simulink model "Crazyflie_NoLinealModel"  (R2020b)
settings: Solver=VariableStepAuto  StartTime=0.0  StopTime=10.0  RelTol=1e-3
undefined symbols (not defined in the file): fm, g, Ixx, Iyy, Izz, m, MNL1
settings Model: Creator=FranciscoJose  LastModifiedBy=FranciscoJose

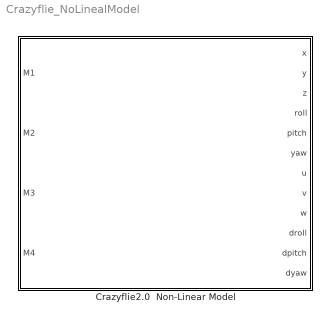
== system Crazyflie_NoLinealModel ==
  Crazyflie2.0  Non-Linear Model : Subsystem
      mask Display: image('crazyflie_icon.png')

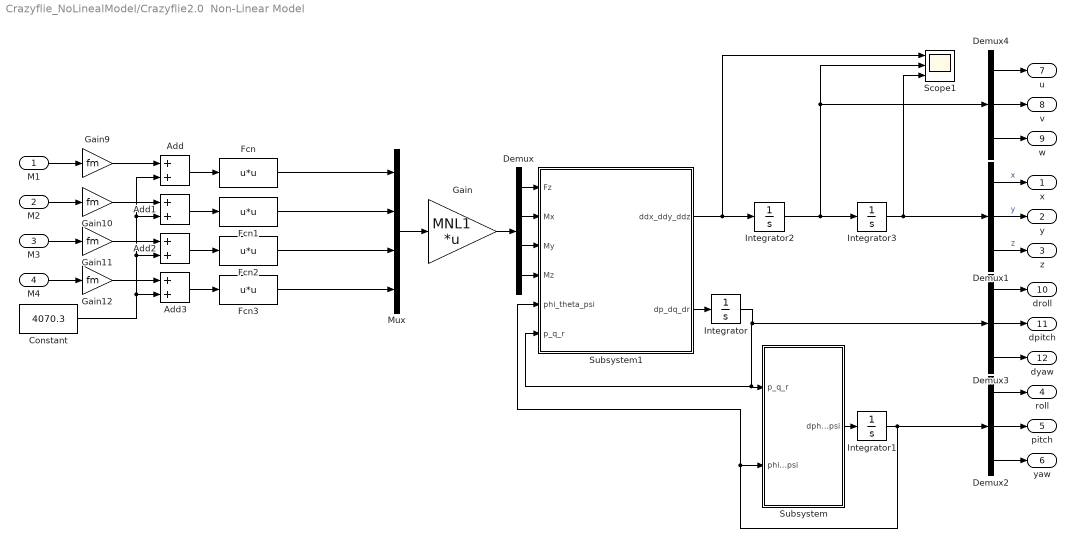
== system Crazyflie_NoLinealModel/Crazyflie2.0  Non-Linear Model ==
  M1 : Inport
  M2 : Inport  Port=2
  M3 : Inport  Port=3
  M4 : Inport  Port=4
  Add{,1..3} (4 alike) : Sum
  Constant : Constant  Value=4070.3
  Demux : Demux
  Demux{1..4} (4 alike) : Demux  Outputs=3
  Fcn{,1..3} (4 alike) : Fcn  Expr=u*u
  Gain : Gain  Gain=MNL1  Multiplication=Matrix(K*u) (u vector)
  Gain{9..12} (4 alike) : Gain  Gain=fm
  Integrator{,1..3} (4 alike) : Integrator
  Mux : Mux
  Scope1 : Scope  NumInputPorts=3
  Subsystem : Subsystem
  Subsystem1 : Subsystem
  x : Outport
  y : Outport  Port=2
  z : Outport  Port=3
  roll : Outport  Port=4
  pitch : Outport  Port=5
  yaw : Outport  Port=6
  u : Outport  Port=7
  v : Outport  Port=8
  w : Outport  Port=9
  droll : Outport  Port=10
  dpitch : Outport  Port=11
  dyaw : Outport  Port=12
  wires:
  Mux/1 -> Gain/1
  Gain/1 -> Demux/1
  Demux/1 -> Subsystem1/1(Fz)
  Demux/2 -> Subsystem1/2(Mx)
  Demux/3 -> Subsystem1/3(My)
  Demux/4 -> Subsystem1/4(Mz)
  Demux1/1 -> x/1  "x"
  Demux1/2 -> y/1  "y"
  Demux1/3 -> z/1  "z"
  Demux2/1 -> roll/1
  Demux2/2 -> pitch/1
  Demux2/3 -> yaw/1
  Demux4/1 -> u/1
  Demux4/2 -> v/1
  Demux4/3 -> w/1
  Demux3/1 -> droll/1
  Demux3/2 -> dpitch/1
  Demux3/3 -> dyaw/1
  M1/1 -> Gain9/1
  M2/1 -> Gain10/1
  M3/1 -> Gain11/1
  M4/1 -> Gain12/1
  Subsystem1/2(dp_dq_dr) -> Integrator/1
  Integrator/1 -> Demux3/1, Subsystem1/6(p_q_r), Subsystem/1(p_q_r)
  Subsystem/1(dphi_dtheta_dpsi) -> Integrator1/1
  Integrator1/1 -> Demux2/1, Subsystem1/5(phi_theta_psi), Subsystem/2(phi_theta_psi)
  Subsystem1/1(ddx_ddy_ddz) -> Scope1/1, Integrator2/1
  Integrator2/1 -> Demux4/1, Scope1/2, Integrator3/1
  Integrator3/1 -> Demux1/1, Scope1/3
  Add/1 -> Fcn/1
  Add1/1 -> Fcn1/1
  Add2/1 -> Fcn2/1
  Add3/1 -> Fcn3/1
  Gain9/1 -> Add/1
  Gain10/1 -> Add1/1
  Gain11/1 -> Add2/1
  Gain12/1 -> Add3/1
  Constant/1 -> Add3/2, Add/2, Add1/2, Add2/2
  Fcn2/1 -> Mux/3
  Fcn/1 -> Mux/1
  Fcn3/1 -> Mux/4
  Fcn1/1 -> Mux/2

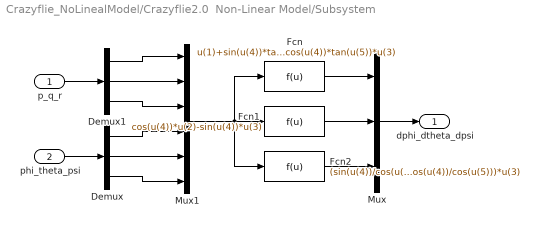
== system Crazyflie_NoLinealModel/Crazyflie2.0  Non-Linear Model/Subsystem ==
  p_q_r : Inport
  phi_theta_psi : Inport  Port=2
  Demux : Demux  Outputs=3
  Demux1 : Demux  Outputs=3
  Fcn : Fcn  Expr=u(1)+sin(u(4))*tan(u(5))*u(2)+cos(u(4))*tan(u(5))*u(3)
  Fcn1 : Fcn  Expr=cos(u(4))*u(2)-sin(u(4))*u(3)
  Fcn2 : Fcn  Expr=(sin(u(4))/cos(u(5)))*u(2)+(cos(u(4))/cos(u(5)))*u(3)
  Mux : Mux  Inputs=3
  Mux1 : Mux  Inputs=6
  dphi_dtheta_dpsi : Outport
  wires:
  Mux1/1 -> Fcn2/1, Fcn/1, Fcn1/1
  Fcn2/1 -> Mux/3
  Fcn/1 -> Mux/1
  Fcn1/1 -> Mux/2
  Mux/1 -> dphi_dtheta_dpsi/1
  Demux/3 -> Mux1/6
  Demux/2 -> Mux1/5
  Demux/1 -> Mux1/4
  Demux1/3 -> Mux1/3
  Demux1/2 -> Mux1/2
  Demux1/1 -> Mux1/1
  phi_theta_psi/1 -> Demux/1
  p_q_r/1 -> Demux1/1

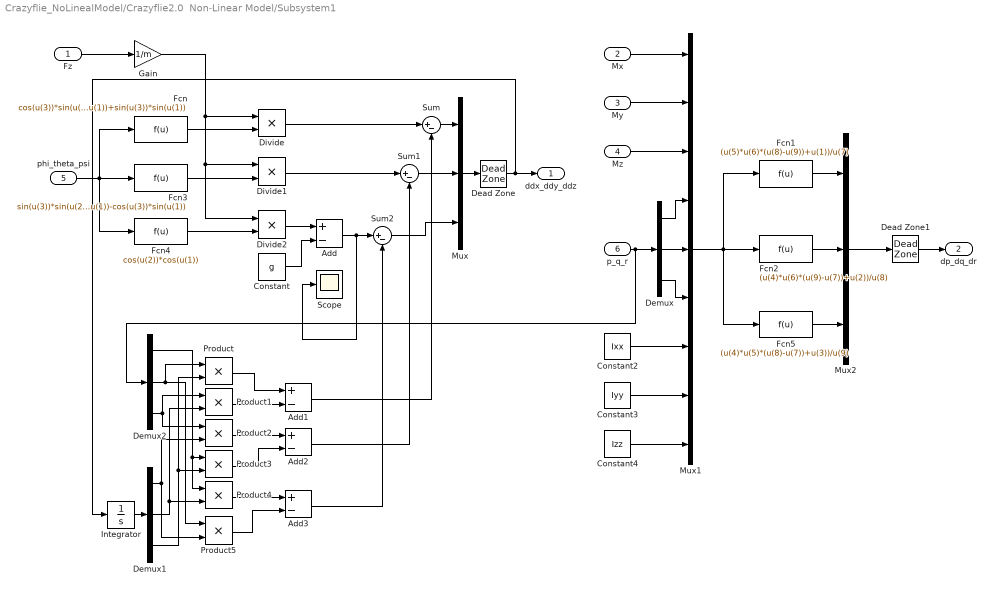
== system Crazyflie_NoLinealModel/Crazyflie2.0  Non-Linear Model/Subsystem1 ==
  Fz : Inport
  Mx : Inport  Port=2
  My : Inport  Port=3
  Mz : Inport  Port=4
  phi_theta_psi : Inport  Port=5
  p_q_r : Inport  Port=6
  Add{,1..3} (4 alike) : Sum  Inputs=+-
  Constant : Constant  Value=g
  Constant2 : Constant  Value=Ixx
  Constant3 : Constant  Value=Iyy
  Constant4 : Constant  Value=Izz
  Dead Zone : DeadZone  LowerValue=-0.0001  UpperValue=0.0001  SaturateOnIntegerOverflow=on
  Dead Zone1 : DeadZone  LowerValue=-0.0001  UpperValue=0.0001  SaturateOnIntegerOverflow=on
  Demux : Demux  Outputs=3
  Demux1 : Demux  Outputs=3
  Demux2 : Demux  Outputs=3
  Divide : Product  Inputs=**
  Divide1 : Product  Inputs=**
  Divide2 : Product  Inputs=**
  Fcn : Fcn  Expr=cos(u(3))*sin(u(2))*cos(u(1))+sin(u(3))*sin(u(1))
  Fcn1 : Fcn  Expr=(u(5)*u(6)*(u(8)-u(9))+u(1))/u(7)
  Fcn2 : Fcn  Expr=(u(4)*u(6)*(u(9)-u(7))+u(2))/u(8)
  Fcn3 : Fcn  Expr=sin(u(3))*sin(u(2))*sin(u(1))-cos(u(3))*sin(u(1))
  Fcn4 : Fcn  Expr=cos(u(2))*cos(u(1))
  Fcn5 : Fcn  Expr=(u(4)*u(5)*(u(8)-u(7))+u(3))/u(9)
  Gain : Gain  Gain=1/m
  Integrator : Integrator
  Mux : Mux  Inputs=3
  Mux1 : Mux  Inputs=9
  Mux2 : Mux  Inputs=3
  Product{,1..5} (6 alike) : Product
  Scope : Scope
  Sum : Sum  Inputs=|+-
  Sum1 : Sum  Inputs=|+-
  Sum2 : Sum  Inputs=|+-
  ddx_ddy_ddz : Outport
  dp_dq_dr : Outport  Port=2
  wires:
  Fz/1 -> Gain/1
  phi_theta_psi/1 -> Fcn/1, Fcn3/1, Fcn4/1
  Fcn/1 -> Divide/2
  Gain/1 -> Divide/1, Divide1/1, Divide2/1
  Fcn3/1 -> Divide1/2
  Fcn4/1 -> Divide2/2
  Divide2/1 -> Add/1
  Constant/1 -> Add/2
  Divide/1 -> Sum/1
  Divide1/1 -> Sum1/1
  Add/1 -> Sum2/1, Scope/1
  p_q_r/1 -> Demux/1, Demux2/1
  Mx/1 -> Mux1/1
  My/1 -> Mux1/2
  Demux/2 -> Mux1/5
  Mz/1 -> Mux1/3
  Demux/1 -> Mux1/4
  Demux/3 -> Mux1/6
  Constant4/1 -> Mux1/9
  Constant3/1 -> Mux1/8
  Constant2/1 -> Mux1/7
  Fcn1/1 -> Mux2/1
  Fcn2/1 -> Mux2/2
  Fcn5/1 -> Mux2/3
  Mux1/1 -> Fcn1/1, Fcn2/1, Fcn5/1
  Mux2/1 -> Dead Zone1/1
  Mux/1 -> Dead Zone/1
  Dead Zone/1 -> ddx_ddy_ddz/1, Integrator/1
  Dead Zone1/1 -> dp_dq_dr/1
  Integrator/1 -> Demux1/1
  Demux2/2 -> Product5/1, Product/1
  Demux1/3 -> Product3/2, Product/2
  Product/1 -> Add1/1
  Demux2/3 -> Product2/1, Product1/1
  Demux1/2 -> Product4/2, Product1/2
  Product1/1 -> Add1/2
  Demux1/1 -> Product5/2, Product2/2
  Product2/1 -> Add2/1
  Demux2/1 -> Product4/1, Product3/1
  Product3/1 -> Add2/2
  Product4/1 -> Add3/1
  Product5/1 -> Add3/2
  Sum/1 -> Mux/1
  Sum1/1 -> Mux/2
  Sum2/1 -> Mux/3
  Add3/1 -> Sum2/2
  Add2/1 -> Sum1/2
  Add1/1 -> Sum/2
